simulink subsystem "MotorOutput"  (R2025a)
settings: Solver=VariableStepAuto  StartTime=0.0  StopTime=10.0  RelTol=1e-3
libraries: arduinoavrlib x4, simulink x2
settings Model: Creator=tobia  LastModifiedBy=tobia

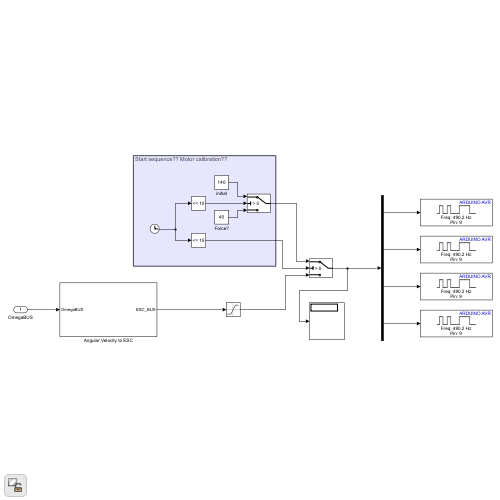
[thumbnail: Simulink's stored preview of the top-level diagram]
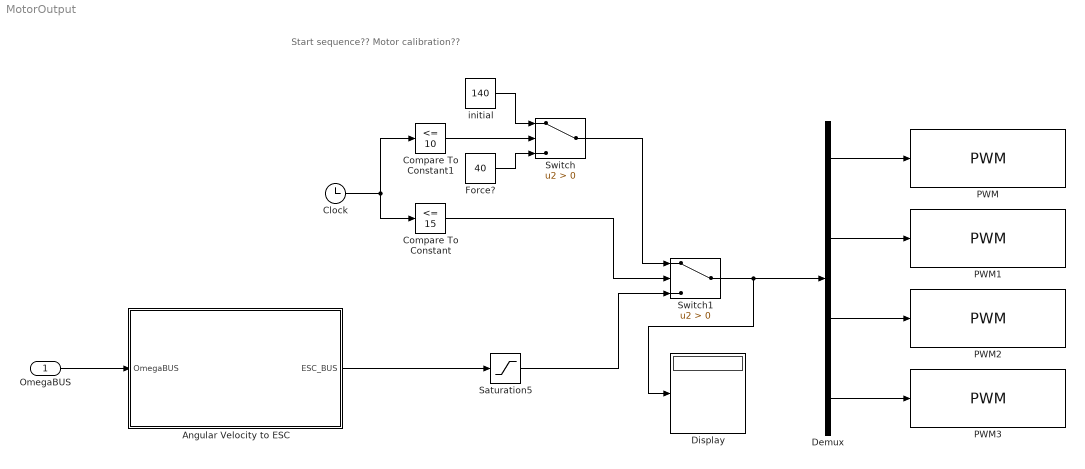
== system MotorOutput ==
  note: Start sequence?? Motor calibration??
  OmegaBUS : Inport
  Angular Velocity to ESC : Subsystem
  Clock : Clock
  Compare To Constant : simulink/Logic and Bit Operations/Compare To Constant  relop=<=  const=15  OutDataTypeStr=boolean
  Compare To Constant1 : simulink/Logic and Bit Operations/Compare To Constant  relop=<=  const=10  OutDataTypeStr=boolean
  Demux : Demux
  Display : Display
  Force? : Constant  Value=40
  PWM{,1..3} (4 alike) : arduinoavrlib/PWM  pinNumber=9  desiredFrequency=490.2  achievableFrequency=490.2  EnableCompareMatchInterrupt=off  EnableOverflowInterrupt=off
  Saturation5 : Saturate  UpperLimit=120  LowerLimit=40
  Switch : Switch  Criteria=u2 > Threshold  SaturateOnIntegerOverflow=off  InputSameDT=off
  Switch1 : Switch  Criteria=u2 > Threshold  SaturateOnIntegerOverflow=off  InputSameDT=off
  initial : Constant  Value=140
  wires:
  Clock/1 -> Compare To Constant/1, Compare To Constant1/1
  Compare To Constant1/1 -> Switch/2
  initial/1 -> Switch/1
  Force?/1 -> Switch/3
  Switch/1 -> Switch1/1
  Compare To Constant/1 -> Switch1/2
  Angular Velocity to ESC/1(ESC_BUS) -> Saturation5/1
  Switch1/1 -> Demux/1, Display/1
  Demux/1 -> PWM/1
  Demux/2 -> PWM1/1
  Demux/3 -> PWM2/1
  Demux/4 -> PWM3/1
  Saturation5/1 -> Switch1/3
  OmegaBUS/1 -> Angular Velocity to ESC/1(OmegaBUS)

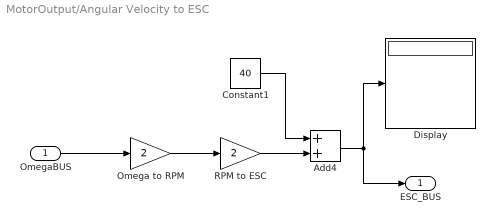
== system MotorOutput/Angular Velocity to ESC ==
  OmegaBUS : Inport
  Add4 : Sum
  Constant1 : Constant  Value=40
  Display : Display
  Omega to RPM : Gain  Gain=2
  RPM to ESC : Gain  Gain=2
  ESC_BUS : Outport
  wires:
  OmegaBUS/1 -> Omega to RPM/1
  RPM to ESC/1 -> Add4/2
  Add4/1 -> Display/1, ESC_BUS/1
  Constant1/1 -> Add4/1
  Omega to RPM/1 -> RPM to ESC/1
